simulink model "pipcontrol"  (Simulink 3.00)
settings: Solver=ode45  SolverMode=SingleTasking  StartTime=0.0  StopTime=10.0  RelTol=1e-3  AbsTol=1e-6
values from neighbouring files (symbols this model uses):
  at = ad    [main_prog.m]    (also in main_prog2.m = Ad)
  bt = bd    [main_prog.m]    (also in main_prog2.m = Bd)
  f = v(1:la)'    [gains.m]
  g = [1 v(la+1:lv-1)']    [gains.m]
  k = v(lv)    [gains.m]
settings Model: LastModifiedBy=kontorou

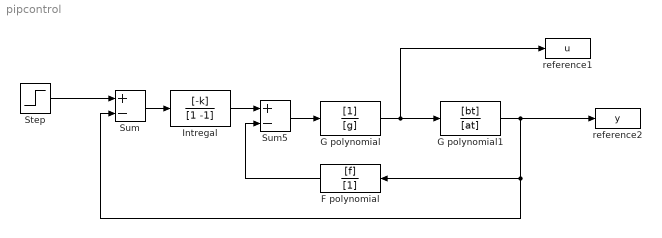
== system pipcontrol ==
  F polynomial : DiscreteFilter  Orientation=left  Numerator=[f]  Denominator=[1]  SampleTime=1
  G polynomial : DiscreteFilter  Numerator=[1]  Denominator=[g]  SampleTime=1
  G polynomial1 : DiscreteFilter  Numerator=[bt]  Denominator=[at]  SampleTime=1
  Intregal : DiscreteFilter  Numerator=[-k]  Denominator=[1 -1]  SampleTime=1
  Step : Step  Time=1  Before=0  After=1  SampleTime=0
  Sum : Sum  Inputs=+-  SaturateOnIntegerOverflow=on
  Sum5 : Sum  Inputs=+-  SaturateOnIntegerOverflow=on
  reference1 : ToWorkspace  VariableName=u  SampleTime=1  SaveFormat=Matrix
  reference2 : ToWorkspace  VariableName=y  SampleTime=1  SaveFormat=Matrix
  wires:
  F polynomial/1 -> Sum5/2
  Sum5/1 -> G polynomial/1
  Intregal/1 -> Sum5/1
  Sum/1 -> Intregal/1
  G polynomial/1 -> G polynomial1/1, reference1/1
  G polynomial1/1 -> F polynomial/1, Sum/2, reference2/1
  Step/1 -> Sum/1
